simulink subsystem "FrictionID"  (R2021a)
settings: Solver=VariableStepAuto  StartTime=0.0  StopTime=10.0  RelTol=1e-3
settings Model: Creator=valen  LastModifiedBy=valen

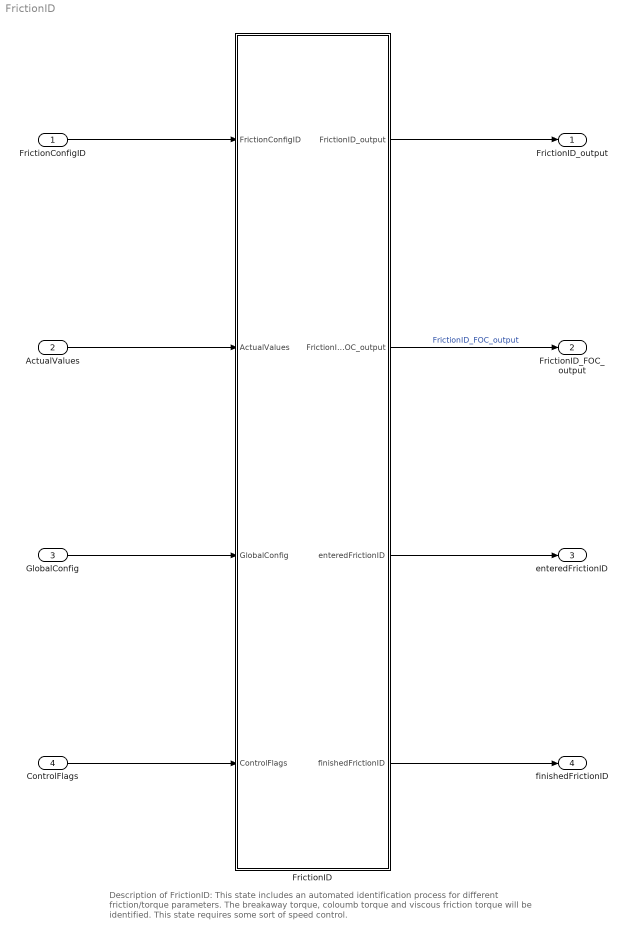
== system FrictionID ==
  note: Description of FrictionID:
      |
      | This state includes an automated identification process for different friction/torque parameters. The breakaway torque, coloumb torque and viscous friction torque will be identified. This state requires some sort of speed control.
  FrictionConfigID : Inport
  ActualValues : Inport  Port=2
  GlobalConfig : Inport  Port=3
  ControlFlags : Inport  Port=4
  FrictionID : Stateflow chart  TreatAsAtomicUnit=on
      settings: PortSchema="{\"entries\":[{\"content\":{\"sides\":[{\"content\":{\"connectorIds\":[\"In1\",\"In2\",\"In3\",\"In4\"]},\"type\":\"ConnectorPlacement.EquallySpacedRectSide\",\"uuid\":\"9228c284-4dde-45fc-9186-6f631f78e5bf\"},{\"content\":{\"connectorIds\":[\"Out4\",\"Out3\",\"Out2\",\"Out1\"],\"side\":\"RIGHT\"},\"type\":\"ConnectorPlacement.EquallySpacedRectSide\",\"uuid\":\"71961043-480b-43aa-8cdd-23d9057d5ad4\"},{\"content\":{\"connectorIds\":[],\"side\":\"TOP\"},\"type\":\"ConnectorPlacement.EquallySpacedRectSide\",\"uuid\":\"f6f3bc9d-566f-4498-bf43-24e8b901b7a7\"}]},\"type\":\"ConnectorPlacement.EquallySpacedConnector\",\"uuid\":\"83d2d7c4-30d1-4ed4-b102-cbae6a0e9817\"}],\"packageUris\":[\"http://schema.mathworks.com/mf0/Connector/R2020b\"],\"version\":\"1.0\"}"
  FrictionID_output : Outport
  FrictionID_FOC_output : Outport  Port=2
  enteredFrictionID : Outport  Port=3
  finishedFrictionID : Outport  Port=4
  wires:
  FrictionID/2(enteredFrictionID) -> enteredFrictionID/1
  GlobalConfig/1 -> FrictionID/3(GlobalConfig)
  FrictionID/4(FrictionID_output) -> FrictionID_output/1
  FrictionID/3(FrictionID_FOC_output) -> FrictionID_FOC_output/1  "FrictionID_FOC_output"
  ControlFlags/1 -> FrictionID/4(ControlFlags)
  ActualValues/1 -> FrictionID/2(ActualValues)
  FrictionID/1(finishedFrictionID) -> finishedFrictionID/1
  FrictionConfigID/1 -> FrictionID/1(FrictionConfigID)

== stateflow chart FrictionID/FrictionID ==
  settings: updateMethod=DISCRETE  sampleTime=1/d_f_states
  note: Friction - identification
  state frictionID
    entry:
    initParams;
    enteredFrictionID=boolean(1);
    FrictionID_FOC_output.activeState=uint16(300);
    during:
    state ResetIntegrator1
      entry:
      counter2=uint32(1);
      FrictionID_FOC_output.activeState=uint16(320);
      during:
      FrictionID_FOC_output.resetIntegrator=boolean(1);
      counter2 = counter2 + 1;
      exit:
      FrictionID_FOC_output.enableFOC_current=boolean(0);
      FrictionID_FOC_output.resetIntegrator=boolean(0);
    state CoulombFrictionTorqueEstimation
      entry:
      FrictionID_FOC_output.activeState = uint16(330);
      FrictionID_FOC_output.enableFOC_speed=boolean(1);
      FrictionID_FOC_output.n_ref_FOC=single(0);
      delay=single(0.1);
      meas_sum=single(zeros(2,1));
      measArray2(1:1024,1:2)=zeros(1024,2);
      omega_Brk=single(5.0);
      nextstate=uint16(0);
      counter=uint32(1);
      mean_count=single(256);
      meas_count=uint16(0);
      during:
      FrictionID_FOC_output.n_ref_FOC=n_eva;
      exit:
      line=gerade;
      FrictionID_output.CoulTorque=single(line(2));
      FrictionID_output.ViscoTorque=single(line(1));
      FrictionID_FOC_output.n_ref_FOC=single(0);
      state SmoothingCurrentAndOmega
        entry: FrictionID_FOC_output.activeState = uint16(331)
        meas_count=uint16(0);
        switcher=boolean(1);
        during:
        if(meas_count==uint32(0.02/GlobalConfig.sampleTimeISR))
        measArray2(mean_count,1)=meas_sum(1)/(0.02/GlobalConfig.sampleTimeISR);
        measArray2(mean_count,2)=meas_sum(2)/(0.02/GlobalConfig.sampleTimeISR);
        meas_sum=single(zeros(2,1));
        if(measArray2(mean_count,1)<((1-FrictionConfigID.eta)*n_eva*0.1047) ||measArray2(mean_count,1)>((1+FrictionConfigID.eta)*n_eva*0.1047))
        switcher=boolean(0);
        end
        mean_count = mean_count + 1;
        meas_count=uint16(0);
        end
        meas_count=meas_count+1;
        meas_sum(1)=meas_sum(1)+abs(ActualValues.omega_m);
        meas_sum(2)=meas_sum(2)+abs(ActualValues.i_dq.q);
      state DecreaseSpeed
        entry:
        counter2 = uint32(1);
        FrictionID_FOC_output.activeState = uint16(332)
        if(n_eva>0&&switcher==boolean(1))
        FrictionID_output.measArraySpeed(counter)=mean(measArray2(1:256,1));
        FrictionID_output.measArrayTorque(counter)=1.5*GlobalConfig.PMSM_config.polePairs*GlobalConfig.PMSM_config.Psi_PM_Vs*mean(measArray2(1:256,2));
        counter=counter+1;
        n_eva=n_eva-(n_eva_step);
        elseif(n_eva>0&&switcher==boolean(0))
        switch_count = switch_count + 1;
        end
        if (n_eva>0 && switch_count>=5)
        n_eva=n_eva-(n_eva_step);
        switch_count = uint32(0);
        end
        if(abs(ActualValues.omega_m)<=omega_Brk&&counter>2)
        n_eva=single(0);
        nextstate=uint16(1);
        end
        during:
        counter2 = counter2 +1;
        exit:
        mean_count=1;
      (default) -> SmoothingCurrentAndOmega
      SmoothingCurrentAndOmega -> DecreaseSpeed : [mean_count==256]
      DecreaseSpeed -> SmoothingCurrentAndOmega : [delay_transition_counter == counter2]
    state BreakawayTorqueEstimation
      entry:
      FrictionID_FOC_output.activeState = uint16(310);
      FrictionID_FOC_output.enableFOC_current=boolean(1);
      FrictionID_FOC_output.resetIntegrator=boolean(0);
      during:
      FrictionID_FOC_output.i_dq_ref.q=i_eva;
      if(nextstate>=FrictionConfigID.BrkCount)
      i_eva=single(0);
      if(counter<=FrictionConfigID.N_Brk)
      Ustep(counter)=i_Brk;
      end
      nextstate=uint16(0);
      counter = counter + 1;
      end
      exit:
      i_Brk=max(Ustep);
      FrictionID_output.BrkTorque=single(3*GlobalConfig.PMSM_config.polePairs*GlobalConfig.PMSM_config.Psi_PM_Vs*i_Brk*0.5);
      state waitstate
        entry:
        counter2 = uint32(1);
        FrictionID_FOC_output.activeState=uint16(311);
        during:
        counter2 = counter2 + 1;
      state increaseCurrent
        entry:
        FrictionID_FOC_output.activeState = uint16(312);
        if(abs(ActualValues.omega_m)>single(0) && i_eva>single(0))
        i_Brk=i_eva;
        nextstate=nextstate+1;
        end
        if(abs(ActualValues.omega_m)<=omega_Brk&&abs(i_eva)<FrictionConfigID.maxCurrent)
        i_eva=i_eva+i_eva_step;
        nextstate=uint16(0);
        end
      (default) -> waitstate
      increaseCurrent -> waitstate
      waitstate -> increaseCurrent : [delay_transition_counter == counter2]
    state FinishDataTransfer
      entry:
      counter2=uint32(1);
      FrictionID_FOC_output.resetIntegrator=boolean(1);
      FrictionID_FOC_output.activeState=uint16(341);
      during:
      counter2 = counter2 +1;
      exit:
      finishedFrictionID=boolean(1);
      enteredFrictionID=boolean(0);
      reset_FOC_output;
    state ResetIntegrator
      entry:
      counter2=uint32(1);
      FrictionID_FOC_output.activeState=uint16(340);
      during:
      counter2 = counter2 +1;
      FrictionID_FOC_output.resetIntegrator=boolean(1);
      exit:
    (default) -> BreakawayTorqueEstimation
    BreakawayTorqueEstimation -> ResetIntegrator1 : [counter>FrictionConfigID.N_Brk]
    ResetIntegrator1 -> CoulombFrictionTorqueEstimation : [one_sec_transition_counter == counter2]
    CoulombFrictionTorqueEstimation -> ResetIntegrator : [nextstate==1]
    ResetIntegrator -> FinishDataTransfer : [ten_sec_transition_counter == counter2]
  state Waiting
    entry:
    %wait for activation of
    %FrictionID
    %donothing
  note: ---
  Waiting -> frictionID [order 1] : [ControlFlags.startFrictionID==1 && GlobalConfig.Reset==0 && GlobalConfig.ACCEPT==1]
  (default) -> Waiting
  Waiting -> Waiting [order 2] : [GlobalConfig.Reset==1]{finishedFrictionID=boolean(0);
      | enteredFrictionID=boolean(0);
      | initParams;}
  frictionID -> Waiting : [GlobalConfig.Reset==1 || GlobalConfig.FrictionID==0 || ....
      | GlobalConfig.enableParameterID==0]
      | {enteredFrictionID=boolean(0);initParams;}
  FinishDataTransfer -> Waiting : [one_sec_transition_counter == counter2]
  data: u function_output single size=[2 1]; counter local; measArray2 local; Ustep local; delay local; i_Brk local; i_eva local; i_eva_step local; line local single size=[2 1]; mean_count local single; meas_count local; meas_sum local; nextstate local; omega_Brk local; switcher local boolean; finishedFrictionID output boolean; enteredFrictionID output boolean; FrictionConfigID input Bus: uz_ParaID_FrictionIDConfig_t; FrictionID_FOC_output output Bus: uz_ParaID_Controller_Parameters_output_t; ActualValues input Bus: uz_ParaID_ActualValues_t; GlobalConfig input Bus: uz_ParaID_GlobalConfig_t; ControlFlags input Bus: uz_ParaID_ControlFlags_t; FrictionID_output output Bus: uz_ParaID_FrictionID_output_t; n_eva_step local; n_eva local; one_sec_transition_counter local; delay_transition_counter local; counter2 local; ten_sec_transition_counter local; switch_count local
  function u=gerade:
    | function u=gerade
    | 
    | %Evaluation of Coulomb and viscous torque 
    | %using a linear regression line
    | 
    | %--------initalizing---------------------------------------
    | gerade=single(zeros(2,1));
    | zaehler=single(0);
    | measSum=single(0);
    | iestSum=single(0);
    | Xy=single(0);
    | Xx=single(0);
    | meanMeas=single(0);
    | meanIest=single(0);
    | SS_xy=single(0);
    | SS_xx=single(0);
    | 
    | %--------summing up----------------------------------
    | for k=single(2):single(255)
    |     
    |     %----------reject outliers---------------------------
    |     if (FrictionID_output.measArraySpeed(k) >5 && ( FrictionID_output.measArrayTorque(k)<1.3*FrictionID_output.measArrayTorque(k+1)....
    |             || FrictionID_output.measArrayTorque(k)<1.3*FrictionID_output.measArrayTorque(k-1) ) &&....
    |             ( FrictionID_output.measArrayTorque(k)>FrictionID_output.measArrayTorque(k+1)*0.7  ||....
    |             FrictionID_output.measArrayTorque(k)>FrictionID_output.measArrayTorque(k-1)*0.7 )  )
    |         zaehler=zaehler+1;
    |         measSum=measSum+FrictionID_output.measArraySpeed(k);
    |         iestSum=iestSum+FrictionID_output.measArrayTorque(k);        
    |         Xy=FrictionID_output.measArraySpeed(k)*FrictionID_output.measArrayTorque(k)+Xy;
    |         Xx=FrictionID_output.measArraySpeed(k)*FrictionID_output.measArraySpeed(k)+Xx;
    |     end
    |        
    | end
    | 
    | %-------calculate mean-------------------------------
    | meanMeas=measSum/zaehler;
    | meanIest=iestSum/zaehler;
    | 
    | %----------calculate varianz--------------------------
    |     SS_xy = Xy-zaehler*meanMeas*meanIest; 
    |     SS_xx = Xx- zaehler*meanMeas*meanMeas; 
    | 
    | %-------viscous friction-------------------------------    
    | gerade(1)=single(SS_xy/SS_xx);
    | 
    | %-------Coulomb friction-----------------------------
    | gerade(2)=single(meanIest-(SS_xy/SS_xx)*meanMeas);
    | 
    | u=gerade;
    | end
  function initParams:
    | function initParams
    | 
    | %This is used instead of "after(1.0,sec) to ensure the same transition time
    | %independelty of the sampletime in the c-code
    | one_sec_transition_counter = uint32(1/GlobalConfig.sampleTimeISR);
    | ten_sec_transition_counter = uint32(10/GlobalConfig.sampleTimeISR);
    | delay_transition_counter = uint32(single(5*(GlobalConfig.Kp_iq / GlobalConfig.Ki_iq))/GlobalConfig.sampleTimeISR);
    | % initialize variables
    | meas_sum            = single(zeros(2,1));
    | measArray2 			= single(zeros(2048,2));
    | counter             = uint32(1);
    | switch_count        = uint32(0);
    | Ustep               = single(zeros(103,1));
    | nextstate           = uint16(0);
    | i_eva               = single(0);
    | n_eva               = single(FrictionConfigID.n_eva_max);
    | n_eva_step          = single(n_eva/single(FrictionConfigID.N_Visco));
    | i_Brk               = single(0);
    | mean_count          = single(0);
    | omega_Brk           = single(1);
    | delay               = single(5*(GlobalConfig.Kp_iq / GlobalConfig.Ki_iq));
    | i_eva_step          = single(GlobalConfig.ratCurrent*FrictionConfigID.StepScale);
    | line                = single(zeros(2,1));
    | 
    | %Outputs
    | FrictionID_FOC_output.n_ref_FOC             = single(0.0);
    | FrictionID_FOC_output.i_dq_ref.d            = single(0.0);
    | FrictionID_FOC_output.i_dq_ref.q            = single(i_eva);
    | FrictionID_FOC_output.i_dq_ref.zero         = single(0.0);
    | FrictionID_FOC_output.enableFOC_speed       = boolean(0);
    | FrictionID_FOC_output.enableFOC_current     = boolean(0);
    | FrictionID_FOC_output.resetIntegrator       = boolean(1);
    | finishedFrictionID                          = boolean(0);
    | FrictionID_FOC_output.Kp_id_out             = single(GlobalConfig.Kp_id);
    | FrictionID_FOC_output.Kp_iq_out             = single(GlobalConfig.Kp_iq);
    | FrictionID_FOC_output.Kp_n_out              = single(GlobalConfig.Kp_n);
    | FrictionID_FOC_output.Ki_id_out             = single(GlobalConfig.Ki_id);
    | FrictionID_FOC_output.Ki_iq_out             = single(GlobalConfig.Ki_iq);
    | FrictionID_FOC_output.Ki_n_out              = single(GlobalConfig.Ki_n);
    | FrictionID_FOC_output.activeState           = uint16(0);
    | 
    | FrictionID_output.BrkTorque                 = single(0.0);
    | FrictionID_output.CoulTorque                = single(0.0);
    | FrictionID_output.ViscoTorque               = single(0.0);
    | FrictionID_output.measArraySpeed			= single(zeros(256,1));
    | FrictionID_output.measArrayTorque           = single(zeros(256,1));
    | end
  function reset_FOC_output:
    | function reset_FOC_output
    | 
    | %Outputs
    | FrictionID_FOC_output.n_ref_FOC             = single(0.0);
    | FrictionID_FOC_output.i_dq_ref.d            = single(0.0);
    | FrictionID_FOC_output.i_dq_ref.q            = single(i_eva);
    | FrictionID_FOC_output.i_dq_ref.zero         = single(0.0);
    | FrictionID_FOC_output.enableFOC_speed       = boolean(0);
    | FrictionID_FOC_output.enableFOC_current     = boolean(0);
    | FrictionID_FOC_output.resetIntegrator       = boolean(1);
    | FrictionID_FOC_output.Kp_id_out             = single(GlobalConfig.Kp_id);
    | FrictionID_FOC_output.Kp_iq_out             = single(GlobalConfig.Kp_iq);
    | FrictionID_FOC_output.Kp_n_out              = single(GlobalConfig.Kp_n);
    | FrictionID_FOC_output.Ki_id_out             = single(GlobalConfig.Ki_id);
    | FrictionID_FOC_output.Ki_iq_out             = single(GlobalConfig.Ki_iq);
    | FrictionID_FOC_output.Ki_n_out              = single(GlobalConfig.Ki_n);
    | FrictionID_FOC_output.activeState               = uint16(0);
    | end
